simulink model "MRAC_CasoEscalar_07_03_2018"  (R2013b)
settings: Solver=ode45  StartTime=0.0  StopTime=50  FixedStep=0.1  RelTol=1e-3
libraries: simulink x1
settings Model: Creator=Eduardo  LastModifiedBy=Eduardo

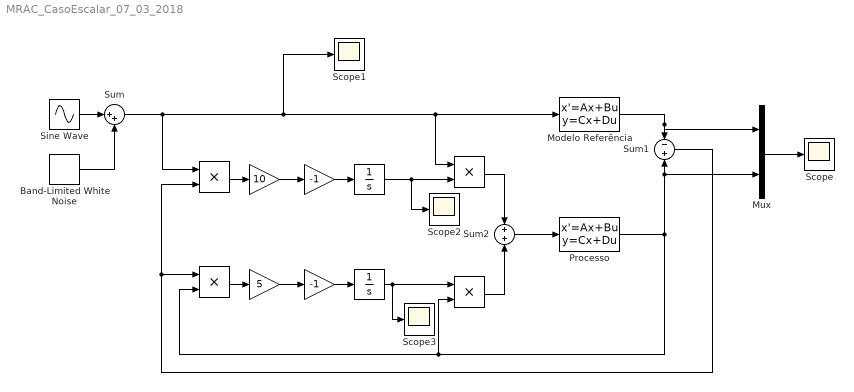
== system MRAC_CasoEscalar_07_03_2018 ==
  " " : Gain  Gain=-1
  "  " : Gain  Gain=-1
  "   " : Integrator
  "     " : Integrator
  "      " : Gain  Gain=10
  "               " : Product
  "                     " : Gain  Gain=5
  "                       " : Product
  "                           " : Product
  "                            " : Product
  Band-Limited White Noise : simulink/Sources/Band-Limited White Noise  Cov=[0.01]  Ts=0.1  seed=[23341]
  "Modelo Referência " : StateSpace  A=-1  D=0  X0=0
  Mux : Mux  Inputs=2
  "Processo " : StateSpace  A=-2  B=0.5  D=0  X0=0
  Scope{,1..3} (4 alike) : Scope
      Scope2 settings: SaveName=ScopeData2
      Scope3 settings: SaveName=ScopeData3
  Sine Wave : Sin  SampleTime=0
  Sum : Sum  Inputs=|++
  Sum1 : Sum  Inputs=-|+
  Sum2 : Sum  Inputs=+|+
  wires:
  Sine Wave/1 -> Sum/1
  Band-Limited White Noise/1 -> Sum/2
  Sum/1 -> Scope1/1, "Modelo Referência "/1, "                            "/1, "               "/1
  "Modelo Referência "/1 -> Mux/1, Sum1/1
  "Processo "/1 -> "                           "/2, "                       "/2, Mux/2, Sum1/2
  Sum1/1 -> "                           "/1, "               "/2
  "               "/1 -> "      "/1
  "                           "/1 -> "                     "/1
  "                     "/1 -> "  "/1
  "      "/1 -> " "/1
  " "/1 -> "   "/1
  "  "/1 -> "     "/1
  "   "/1 -> Scope2/1, "                            "/2
  "     "/1 -> "                       "/1, Scope3/1
  "                            "/1 -> Sum2/1
  "                       "/1 -> Sum2/2
  Sum2/1 -> "Processo "/1
  Mux/1 -> Scope/1
